simulink model "PV_DCDC_pretvarac_baterija_i_trosilo_regulator_2019"  (R2023b)
settings: Solver=ode23t  StartTime=14*3600-25  StopTime=14*3600+25  MaxStep=1e-3  RelTol=1e-3  EnableMultiTasking=on
undefined symbols (not defined in the file or in its folder): KRI, KRU1, KRUPV, mppt, pv_data, pv_eq, TII, TIU1, TIUPV
settings Model: Creator=Mario  LastModifiedBy=teo
settings SolverCC: ZeroCrossControl=EnableAll  ZeroCrossAlgorithm=Adaptive  AlgebraicLoopSolver=TrustRegion
settings DataIOCC: LimitDataPoints=on  SaveFormat=Array  SignalLoggingSaveFormat=ModelDataLogs  ReturnWorkspaceOutputs=off
settings OptimizationCC: ExpressionDepthLimit=2147483647  LifeSpan=inf
settings DebuggingCC: UnderspecifiedInitializationDetection=Classic  MergeDetectMultiDrivingBlocksExec=none  SolverPrmCheckMsg=warning  FcnCallInpInsideContextMsg=warning  UnconnectedInputMsg=warning  UnconnectedOutputMsg=warning  UnconnectedLineMsg=warning  StateNameClashWarn=warning  SFUnexpectedBacktrackingDiag=warning  SFNoUnconditionalDefaultTransitionDiag=warning  SFExecutionAtInitializationDiag=none  ArithmeticOperatorsInVariantConditions=warning
settings HardwareCC: ProdBitPerPointer=32  ProdBitPerSizeT=32  ProdBitPerPtrDiffT=32  ProdLargestAtomicFloat=None  ProdIntDivRoundTo=Undefined  ProdEndianess=Unspecified  ProdWordSize=32  ProdHWDeviceType=32-bit Generic
settings ModelReferenceCC: EnableRefExpFcnMdlSchedulingChecks=on  PropagateSignalLabelsOutOfModel=off
settings SFSimCC: SimUseLocalCustomCode=off  CustomCodeUndefinedFunction=UseInterfaceOnly
settings RTWCC: RTWUseLocalCustomCode=off
settings CodeAppCC: StateflowObjectComments=on
settings GRTTargetCC: TargetLangStandard=C89/C90 (ANSI)  CombineOutputUpdateFcns=off  GRTInterface=on
settings ConfigComp: CovMetricSettings=dw  CovSaveCumulativeToWorkspaceVar=on  CovSaveSingleToWorkspaceVar=on  CovExternalEMLEnable=off

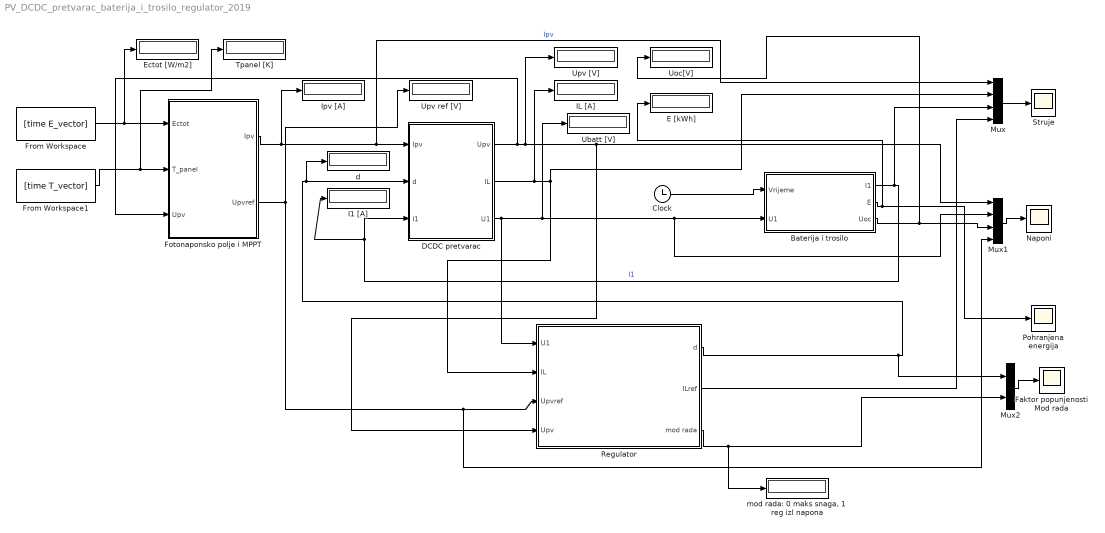
== system PV_DCDC_pretvarac_baterija_i_trosilo_regulator_2019 ==
  Baterija i trosilo : Subsystem
  Clock : Clock
  DCDC pretvarac : Subsystem
  E [kWh] : Display
  Ectot [W/m2] : Display
  Faktor popunjenosti Mod rada : Scope
  Fotonaponsko polje i MPPT : Subsystem
  From Workspace : FromWorkspace  VariableName=[time E_vector]  SampleTime=1  OutputAfterFinalValue=Holding final value
  From Workspace1 : FromWorkspace  VariableName=[time T_vector]  SampleTime=1  OutputAfterFinalValue=Holding final value
  I1 [A] : Display
  IL [A] : Display
  Ipv [A] : Display
  Mux : Mux
  Mux1 : Mux
  Mux2 : Mux  Inputs=2
  Naponi : Scope
  Pohranjena energija : Scope
  Regulator : Subsystem
  Struje : Scope
  Tpanel [K] : Display
  Ubatt [V] : Display
  Uoc[V] : Display
  Upv [V] : Display
  Upv ref [V] : Display
  "d " : Display
  "mod rada: 0 maks snaga, 1 reg izl napona" : Display
  wires:
  Fotonaponsko polje i MPPT/1(Ipv) -> Ipv [A]/1, DCDC pretvarac/1(Ipv), Mux/1  "Ipv"
  DCDC pretvarac/1(Upv) -> Regulator/4(Upv), Mux1/1, Upv [V]/1, Fotonaponsko polje i MPPT/3(Upv)
  From Workspace/1 -> Fotonaponsko polje i MPPT/1(Ectot), Ectot [W/m2]/1
  From Workspace1/1 -> Fotonaponsko polje i MPPT/2(T_panel), Tpanel [K]/1
  DCDC pretvarac/2(IL) -> Regulator/2(IL), Mux/2, IL [A]/1
  DCDC pretvarac/3(U1) -> Regulator/1(U1), Baterija i trosilo/2(U1), Mux1/2, Ubatt [V]/1
  Baterija i trosilo/2(E) -> Pohranjena energija/1, E [kWh]/1
  Clock/1 -> Baterija i trosilo/1(Vrijeme)
  Baterija i trosilo/1(I1) -> DCDC pretvarac/3(I1), I1 [A]/1, Mux/3  "I1"
  Regulator/1(d) -> Mux2/1, DCDC pretvarac/2(d), "d "/1
  Fotonaponsko polje i MPPT/2(Upvref) -> Regulator/3(Upvref), Mux1/4, Upv ref [V]/1
  Mux/1 -> Struje/1
  Mux1/1 -> Naponi/1
  Baterija i trosilo/3(Uoc) -> Mux1/3, Uoc[V]/1
  Mux2/1 -> Faktor popunjenosti Mod rada/1
  Regulator/3(mod rada) -> Mux2/2, "mod rada: 0 maks snaga, 1 reg izl napona"/1
  Regulator/2(ILref) -> Mux/4

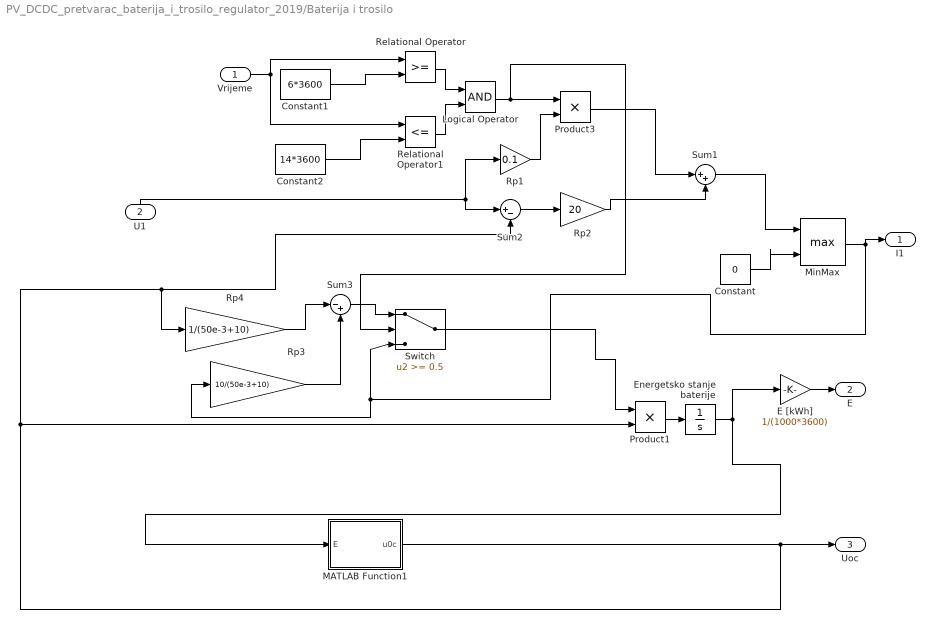
== system PV_DCDC_pretvarac_baterija_i_trosilo_regulator_2019/Baterija i trosilo ==
  Vrijeme : Inport
  U1 : Inport  Port=2
  Constant : Constant  Value=0
  Constant1 : Constant  Value=6*3600
  Constant2 : Constant  Value=14*3600
  E [kWh] : Gain  Gain=1/(1000*3600)
  Energetsko stanje baterije : Integrator  InitialCondition=5000*3600  LimitOutput=on  UpperSaturationLimit=10000*3600  LowerSaturationLimit=0
  Logical Operator : Logic  AllPortsSameDT=off  OutDataTypeStr=boolean
  MATLAB Function1 : MATLAB Function  TreatAsAtomicUnit=on
  MinMax : MinMax  Function=max  Inputs=2
  Product1 : Product
  Product3 : Product
  Relational Operator : RelationalOperator  OutDataTypeStr=boolean  InputSameDT=off
  Relational Operator1 : RelationalOperator  Operator=<=  OutDataTypeStr=boolean  InputSameDT=off
  Rp1 : Gain  Gain=0.1
  Rp2 : Gain  Gain=20
  Rp3 : Gain  Gain=10/(50e-3+10)
  Rp4 : Gain  Gain=1/(50e-3+10)
  Sum1 : Sum  Inputs=|++
  Sum2 : Sum  Inputs=|+-
  Sum3 : Sum  Inputs=|-+
  Switch : Switch  Threshold=0.5  SaturateOnIntegerOverflow=off  InputSameDT=off
  I1 : Outport
  E : Outport  Port=2
  Uoc : Outport  Port=3
  wires:
  Sum3/1 -> Switch/1
  Rp4/1 -> Sum3/1
  Rp3/1 -> Sum3/2
  Product3/1 -> Sum1/1
  Rp2/1 -> Sum1/2
  Sum2/1 -> Rp2/1
  Rp1/1 -> Product3/2
  Logical Operator/1 -> Product3/1, Switch/2
  Relational Operator1/1 -> Logical Operator/2
  Relational Operator/1 -> Logical Operator/1
  Vrijeme/1 -> Relational Operator/1, Relational Operator1/1
  Constant2/1 -> Relational Operator1/2
  Constant1/1 -> Relational Operator/2
  Sum1/1 -> MinMax/1
  Constant/1 -> MinMax/2
  MinMax/1 -> Switch/3, Rp3/1, I1/1
  U1/1 -> Sum2/1, Rp1/1
  Energetsko stanje baterije/1 -> E [kWh]/1, MATLAB Function1/1(E)
  Product1/1 -> Energetsko stanje baterije/1
  Switch/1 -> Product1/1
  MATLAB Function1/1(u0c) -> Product1/2, Sum2/2, Rp4/1, Uoc/1
  E [kWh]/1 -> E/1

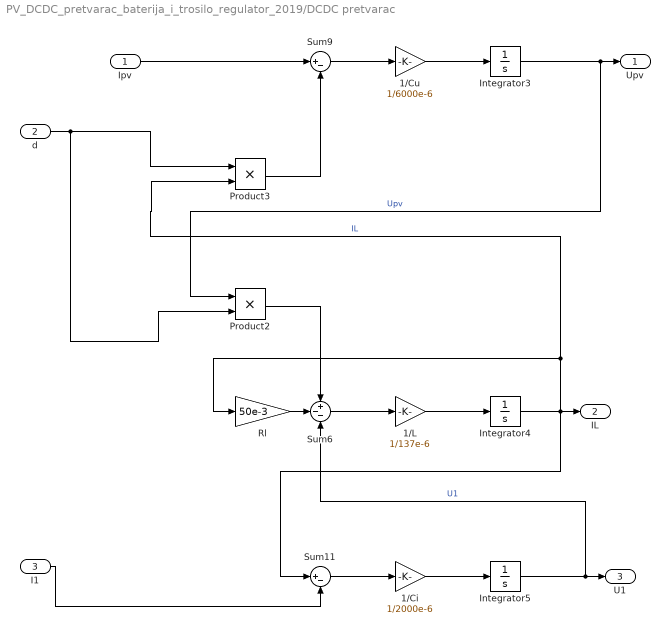
== system PV_DCDC_pretvarac_baterija_i_trosilo_regulator_2019/DCDC pretvarac ==
  Ipv : Inport
  d : Inport  Port=2
  I1 : Inport  Port=3
  1/Ci : Gain  Gain=1/2000e-6
  1/Cu : Gain  Gain=1/6000e-6
  1/L : Gain  Gain=1/137e-6
  Integrator3 : Integrator
  Integrator4 : Integrator
  Integrator5 : Integrator
  Product2 : Product
  Product3 : Product
  Rl : Gain  Gain=50e-3
  Sum11 : Sum  Inputs=|+-
  Sum6 : Sum  Inputs=+--
  Sum9 : Sum  Inputs=|+-
  Upv : Outport
  IL : Outport  Port=2
  U1 : Outport  Port=3
  wires:
  1/Cu/1 -> Integrator3/1
  Integrator3/1 -> Product2/1, Upv/1  "Upv"
  Product2/1 -> Sum6/1
  Sum6/1 -> 1/L/1
  1/L/1 -> Integrator4/1
  Integrator4/1 -> Product3/2, Rl/1, Sum11/1, IL/1  "IL"
  Product3/1 -> Sum9/2
  Sum9/1 -> 1/Cu/1
  1/Ci/1 -> Integrator5/1
  Sum11/1 -> 1/Ci/1
  Rl/1 -> Sum6/2
  Integrator5/1 -> Sum6/3, U1/1  "U1"
  d/1 -> Product3/1, Product2/2
  Ipv/1 -> Sum9/1
  I1/1 -> Sum11/2

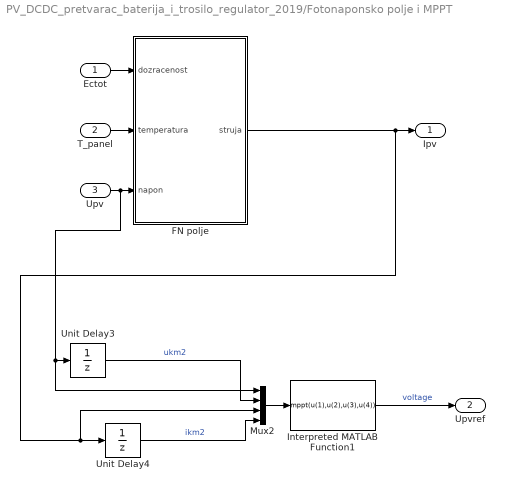
== system PV_DCDC_pretvarac_baterija_i_trosilo_regulator_2019/Fotonaponsko polje i MPPT ==
  Ectot : Inport
  T_panel : Inport  Port=2
  Upv : Inport  Port=3
  FN polje : Subsystem
  Interpreted MATLAB Function1 : MATLABFcn  MATLABFcn=mppt(u(1),u(2),u(3),u(4))  OutputDimensions=1  OutputSignalType=real  Output1D=off  SampleTime=0.1
  Mux2 : Mux
  Unit Delay3 : UnitDelay  SampleTime=0.1
  Unit Delay4 : UnitDelay  SampleTime=0.1
  Ipv : Outport
  Upvref : Outport  Port=2
  wires:
  FN polje/1(struja) -> Ipv/1, Unit Delay4/1, Mux2/3
  Mux2/1 -> Interpreted MATLAB Function1/1
  Interpreted MATLAB Function1/1 -> Upvref/1  "voltage"
  Unit Delay4/1 -> Mux2/4  "ikm2"
  Ectot/1 -> FN polje/1(dozracenost)
  T_panel/1 -> FN polje/2(temperatura)
  Upv/1 -> FN polje/3(napon), Unit Delay3/1, Mux2/1
  Unit Delay3/1 -> Mux2/2  "ukm2"

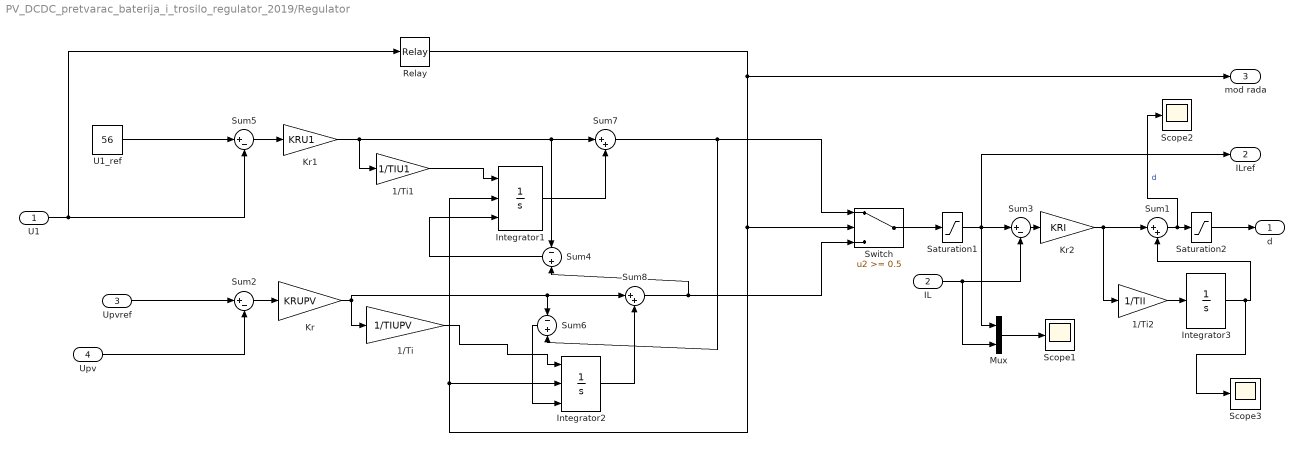
== system PV_DCDC_pretvarac_baterija_i_trosilo_regulator_2019/Regulator ==
  U1 : Inport
  IL : Inport  Port=2
  Upvref : Inport  Port=3
  Upv : Inport  Port=4
  1/Ti : Gain  Gain=1/TIUPV
  1/Ti1 : Gain  Gain=1/TIU1
  1/Ti2 : Gain  Gain=1/TII
  Integrator1 : Integrator  ExternalReset=rising  InitialConditionSource=external  LimitOutput=on  UpperSaturationLimit=50  LowerSaturationLimit=-50
  Integrator2 : Integrator  ExternalReset=falling  InitialConditionSource=external  LimitOutput=on  UpperSaturationLimit=50  LowerSaturationLimit=-50
  Integrator3 : Integrator  LimitOutput=on  UpperSaturationLimit=1  LowerSaturationLimit=0
  Kr : Gain  Gain=KRUPV
  Kr1 : Gain  Gain=KRU1
  Kr2 : Gain  Gain=KRI
  Mux : Mux  Inputs=2
  Relay : Relay  OnSwitchValue=56.2  OffSwitchValue=55.8
  Saturation1 : Saturate  UpperLimit=50  LowerLimit=0
  Saturation2 : Saturate  UpperLimit=1  LowerLimit=0
  Scope1 : Scope
  Scope2 : Scope
  Scope3 : Scope
  Sum1 : Sum  Inputs=|++
  Sum2 : Sum  Inputs=|+-
  Sum3 : Sum  Inputs=|+-
  Sum4 : Sum  Inputs=-|+
  Sum5 : Sum  Inputs=|+-
  Sum6 : Sum  Inputs=-|+
  Sum7 : Sum  Inputs=|++
  Sum8 : Sum  Inputs=|++
  Switch : Switch  Threshold=0.5  SaturateOnIntegerOverflow=off  InputSameDT=off
  U1_ref : Constant  Value=56
  d : Outport
  ILref : Outport  Port=2
  mod rada : Outport  Port=3
  wires:
  Sum3/1 -> Kr2/1
  U1_ref/1 -> Sum5/1
  Switch/1 -> Saturation1/1
  Sum5/1 -> Kr1/1
  Kr1/1 -> 1/Ti1/1, Sum7/1, Sum4/1
  Integrator1/1 -> Sum7/2
  Sum7/1 -> Switch/1, Sum6/2
  Kr/1 -> 1/Ti/1, Sum8/1, Sum6/1
  Sum2/1 -> Kr/1
  Sum8/1 -> Sum4/2, Switch/3
  Integrator2/1 -> Sum8/2
  Saturation1/1 -> Sum3/1, ILref/1, Mux/1
  Upvref/1 -> Sum2/1
  Upv/1 -> Sum2/2
  U1/1 -> Relay/1, Sum5/2
  Relay/1 -> Integrator2/2, Integrator1/2, Switch/2, mod rada/1
  IL/1 -> Sum3/2, Mux/2
  Sum4/1 -> Integrator1/3
  Sum6/1 -> Integrator2/3
  Kr2/1 -> Sum1/1, 1/Ti2/1
  Sum1/1 -> Scope2/1, Saturation2/1  "d"
  1/Ti2/1 -> Integrator3/1
  Integrator3/1 -> Sum1/2, Scope3/1
  Saturation2/1 -> d/1
  1/Ti/1 -> Integrator2/1
  1/Ti1/1 -> Integrator1/1
  Mux/1 -> Scope1/1

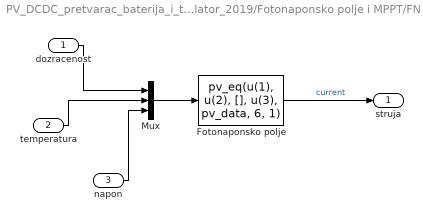
== system PV_DCDC_pretvarac_baterija_i_trosilo_regulator_2019/Fotonaponsko polje i MPPT/FN polje ==
  dozracenost : Inport
  temperatura : Inport  Port=2
  napon : Inport  Port=3
  Fotonaponsko polje : MATLABFcn  MATLABFcn=pv_eq(u(1), u(2), [], u(3), pv_data, 6, 1)  OutputDimensions=1
  Mux : Mux  Inputs=3
  struja : Outport
  wires:
  Mux/1 -> Fotonaponsko polje/1
  dozracenost/1 -> Mux/1
  Fotonaponsko polje/1 -> struja/1  "current"
  temperatura/1 -> Mux/2
  napon/1 -> Mux/3

== matlab function PV_DCDC_pretvarac_baterija_i_trosilo_regulator_2019/Baterija i trosilo/MATLAB Function1 ==
  data: E input; u0c output
function u0c = fcn(E)
%#eml

u0c = 1.4*E/(1000*3600)+42;
